simulink model "iface"  (R2018b)
settings: Solver=FixedStepDiscrete  StartTime=0.0  StopTime=10.0  RelTol=1e-3
settings Model: Creator=matlab  LastModifiedBy=matlab

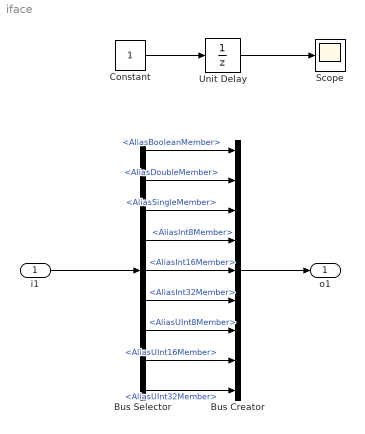
== system iface ==
  i1 : Inport  OutDataTypeStr=Bus: BusDef
  Bus Creator : BusCreator  Inputs=9  OutDataTypeStr=Bus: BusDef  NonVirtualBus=on
  Bus Selector : BusSelector  OutputSignals=AliasBooleanMember,AliasDoubleMember,AliasSingleMember,AliasInt8Member,AliasInt16Member,AliasInt32Member,AliasUInt8Member,AliasUInt16Member,AliasUInt32Member
  Constant : Constant
  Scope : Scope
  Unit Delay : UnitDelay  SampleTime=-1
  o1 : Outport  OutDataTypeStr=Bus: BusDef
  wires:
  Bus Creator/1 -> o1/1
  i1/1 -> Bus Selector/1
  Unit Delay/1 -> Scope/1
  Constant/1 -> Unit Delay/1
  Bus Selector/1 -> Bus Creator/1  "<AliasBooleanMember>"
  Bus Selector/2 -> Bus Creator/2  "<AliasDoubleMember>"
  Bus Selector/3 -> Bus Creator/3  "<AliasSingleMember>"
  Bus Selector/4 -> Bus Creator/4  "<AliasInt8Member>"
  Bus Selector/5 -> Bus Creator/5  "<AliasInt16Member>"
  Bus Selector/6 -> Bus Creator/6  "<AliasInt32Member>"
  Bus Selector/7 -> Bus Creator/7  "<AliasUInt8Member>"
  Bus Selector/8 -> Bus Creator/8  "<AliasUInt16Member>"
  Bus Selector/9 -> Bus Creator/9  "<AliasUInt32Member>"
